simulink model "RegulatorPoPoremecaju"  (Simulink 9.1)
settings: Solver=VariableStepAuto  StartTime=0.0  StopTime=100  RelTol=1e-3
settings Model: Creator=User  LastModifiedBy=User
settings DataIOCC: SaveFormat=Dataset
settings OptimizationCC: LifeSpan=auto
settings DebuggingCC: UnderspecifiedInitializationDetection=Simplified  MergeDetectMultiDrivingBlocksExec=error  SFUnexpectedBacktrackingDiag=error  SFNoUnconditionalDefaultTransitionDiag=error  SFExecutionAtInitializationDiag=warning
settings HardwareCC: ProdBitPerPointer=64  ProdBitPerSizeT=64  ProdBitPerPtrDiffT=64  ProdLargestAtomicFloat=Float  ProdIntDivRoundTo=Zero  ProdEndianess=LittleEndian  ProdWordSize=64  ProdHWDeviceType=Intel->x86-64 (Windows64)
settings ModelReferenceCC: PropagateSignalLabelsOutOfModel=on
settings CodeAppCC: StateflowObjectComments=off
settings GRTTargetCC: TargetLangStandard=C99 (ISO)  CombineOutputUpdateFcns=on  GRTInterface=off
settings ConfigComp: CovMetricSettings=dwe  CovHtmlReporting=off  CovSaveCumulativeToWorkspaceVar=off  CovSaveSingleToWorkspaceVar=off  CovExternalEMLEnable=on

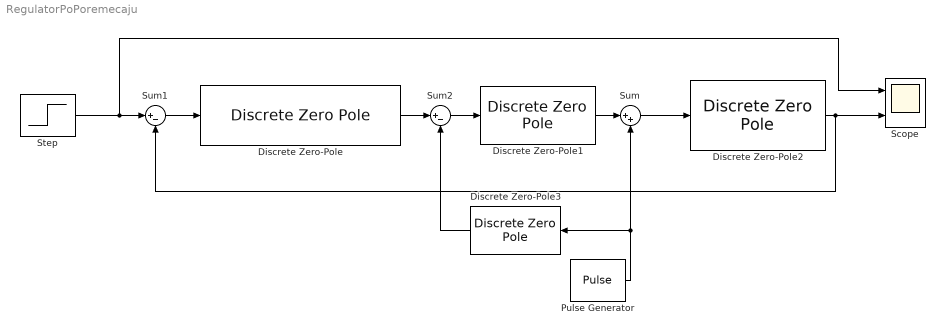
== system RegulatorPoPoremecaju ==
  Discrete Zero-Pole : DiscreteZeroPole  Zeros=[0.7408 0.9306]  Poles=[0.3148 0.985]  Gain=14.2909  SampleTime=0.1
  Discrete Zero-Pole1 : DiscreteZeroPole  Zeros=[-0.8752]  Poles=[0.9048]  Gain=1  SampleTime=0.1
  Discrete Zero-Pole2 : DiscreteZeroPole  Zeros=[]  Poles=[0.7408]  Gain=0.013153  SampleTime=0.1
  Discrete Zero-Pole3 : DiscreteZeroPole  Zeros=[0.9048]  Poles=[-0.8752]  Gain=1  SampleTime=0.1
  Pulse Generator : DiscretePulseGenerator  PulseType=Time based  Amplitude=5  Period=50  PulseWidth=5
  Scope : Scope  NumInputPorts=2
  Step : Step  SampleTime=0
  Sum : Sum  Inputs=|++
  Sum1 : Sum  Inputs=|+-
  Sum2 : Sum  Inputs=|+-
  wires:
  Step/1 -> Scope/1, Sum1/1
  Sum1/1 -> Discrete Zero-Pole/1
  Discrete Zero-Pole1/1 -> Sum/1
  Sum/1 -> Discrete Zero-Pole2/1
  Discrete Zero-Pole2/1 -> Sum1/2, Scope/2
  Pulse Generator/1 -> Sum/2, Discrete Zero-Pole3/1
  Discrete Zero-Pole/1 -> Sum2/1
  Sum2/1 -> Discrete Zero-Pole1/1
  Discrete Zero-Pole3/1 -> Sum2/2
